simulink model "emb_ex_n1_g6"  (R2022a)
settings: Solver=VariableStepAuto  StartTime=0.0  StopTime=10.0  RelTol=1e-3
settings Model: Creator=hora_  LastModifiedBy=hora_

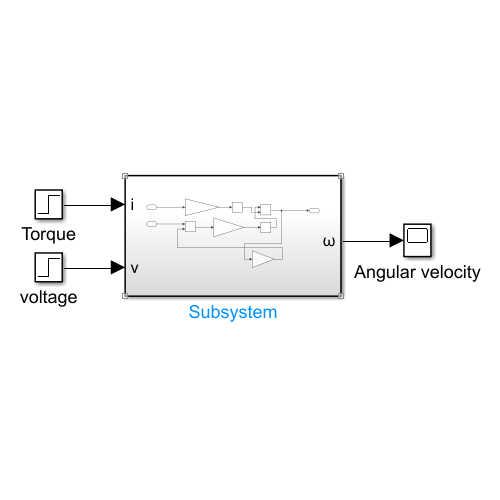
[thumbnail: Simulink's stored preview of the top-level diagram]
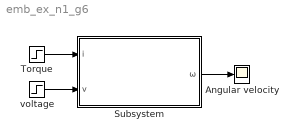
== system emb_ex_n1_g6 ==
  Angular velocity : Scope
  Subsystem : Subsystem
  Torque : Step  Time=5  After=0.01  SampleTime=0
  voltage : Step  Time=0  After=5  SampleTime=0
  wires:
  Torque/1 -> Subsystem/1(i)
  voltage/1 -> Subsystem/2(v)
  Subsystem/1(ω) -> Angular velocity/1

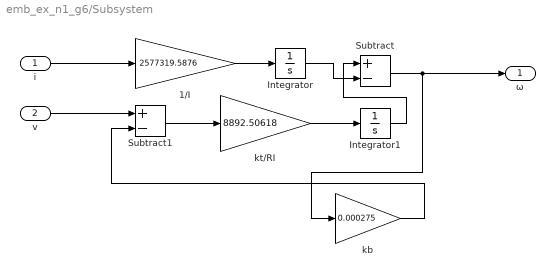
== system emb_ex_n1_g6/Subsystem ==
  i : Inport
  v : Inport  Port=2
  1/I : Gain  Gain=2577319.5876
  Integrator : Integrator
  Integrator1 : Integrator
  Subtract : Sum  Inputs=+-
  Subtract1 : Sum  Inputs=+-
  kb : Gain  Gain=0.000275
  kt/RI : Gain  Gain=8892.50618
  ω : Outport
  wires:
  i/1 -> 1/I/1
  v/1 -> Subtract1/1
  Subtract1/1 -> kt/RI/1
  Subtract/1 -> kb/1, ω/1
  kb/1 -> Subtract1/2
  1/I/1 -> Integrator/1
  Integrator/1 -> Subtract/2
  kt/RI/1 -> Integrator1/1
  Integrator1/1 -> Subtract/1
